simulink model "CK"  (R2023a)
settings: Solver=ode45  StartTime=0.0  StopTime=1000  RelTol=1e-3
values from neighbouring files (symbols this model uses):
  a0 = 0.01    [script.m]
  a1 = 5    [script.m]
  a2 = 10    [script.m]
  Alpha = 1    [script.m]
  b0 = 0.025    [script.m]
  b1 = 0.25    [script.m]
  b2 = 1    [script.m]
  c0 = 0.5    [script.m]
  c1 = 5    [script.m]
  Cyt = 1    [script.m]
  d1 = 1    [script.m]
  k1 = 0.025    [script.m]
  K1 = 1    [script.m]
  K2 = 1    [script.m]
  k2 = 0.5    [script.m]
  Kh1 = 5    [script.m]
  Kh2 = 5    [script.m]
  n = 2    [script.m]
  r1 = 0.025    [script.m]
  r2 = 0.025    [script.m]
  r3 = 0.025    [script.m]
  r4 = 0.025    [script.m]
  V1 = 1    [script.m]
  Vh1 = 2    [script.m]
settings Model: Creator=mosuk  LastModifiedBy=mosuk
settings DataIOCC: ReturnWorkspaceOutputs=off

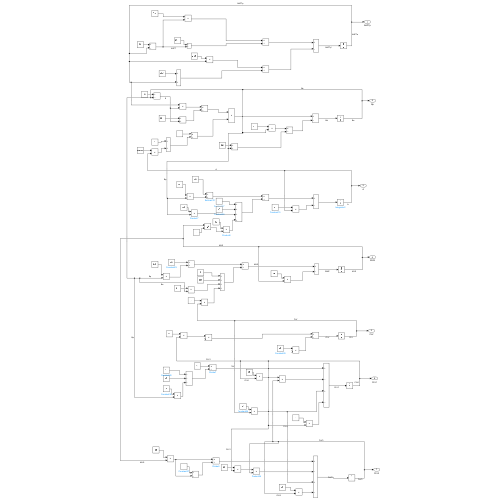
[thumbnail: Simulink's stored preview of the top-level diagram]
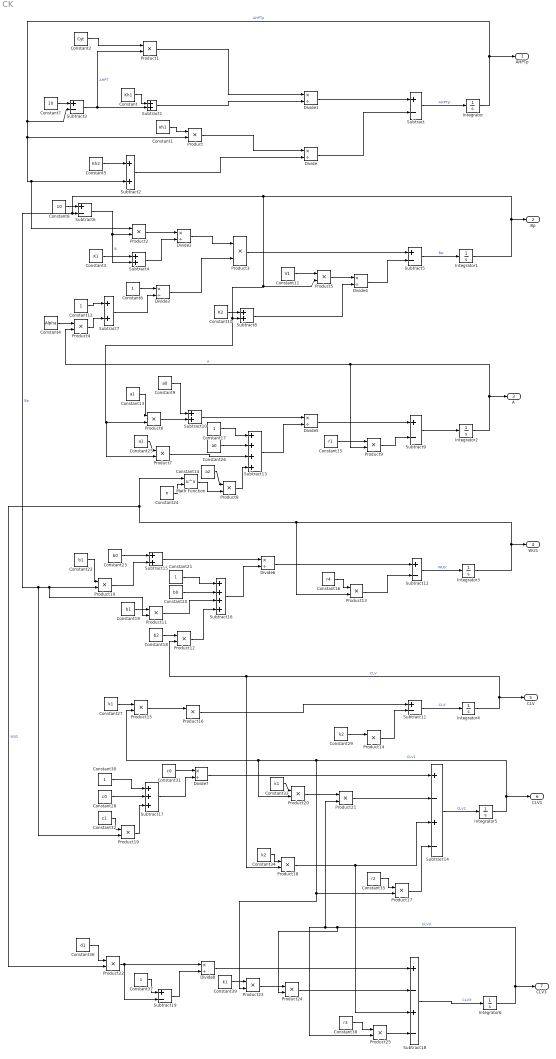
== system CK ==
  Constant : Constant  Value=Kh1
  Constant1 : Constant  Value=Vh1
  Constant10 : Constant  Value=K2
  Constant11 : Constant  Value=V1
  Constant{6,12,17,21,30,37} (6 alike) : Constant
  Constant13 : Constant  Value=a1
  Constant14 : Constant  Value=a2
  Constant15 : Constant  Value=r1
  Constant16 : Constant  Value=r4
  Constant18 : Constant  Value=b2
  Constant19 : Constant  Value=b1
  Constant2 : Constant  Value=Cyt
  Constant20 : Constant  Value=b0
  Constant22 : Constant  Value=b1
  Constant23 : Constant  Value=b0
  Constant24 : Constant  Value=n
  Constant25 : Constant  Value=a1
  Constant26 : Constant  Value=a0
  Constant27 : Constant  Value=k1
  Constant28 : Constant  Value=c0
  Constant29 : Constant  Value=k2
  Constant3 : Constant  Value=K1
  Constant31 : Constant  Value=c0
  Constant32 : Constant  Value=c1
  Constant33 : Constant  Value=k1
  Constant34 : Constant  Value=k2
  Constant35 : Constant  Value=r2
  Constant36 : Constant  Value=d1
  Constant38 : Constant  Value=r3
  Constant39 : Constant  Value=k1
  Constant4 : Constant  Value=Alpha
  Constant5 : Constant  Value=Kh2
  Constant7 : Constant  Value=10
  Constant8 : Constant  Value=10
  Constant9 : Constant  Value=a0
  Divide{,1..8} (9 alike) : Product  Inputs=*/
  Integrator{,1..6} (7 alike) : Integrator
  Math Function : Math  Operator=pow
  Product{,1..25} (26 alike) : Product
  Subtract{,3,5..6,9,11..12,19} (8 alike) : Sum  Inputs=+-
  Subtract{1..2,4,7..8,10,15} (7 alike) : Sum
  Subtract13 : Sum  Inputs=++++
  Subtract14 : Sum  Inputs=+-+-
  Subtract16 : Sum  Inputs=++++
  Subtract17 : Sum  Inputs=+++
  Subtract18 : Sum  Inputs=+-+-
  AHPTp : Outport
  Bp : Outport  Port=2
  A : Outport  Port=3
  WUS : Outport  Port=4
  CLV : Outport  Port=5
  CLV1 : Outport  Port=6
  CLV3 : Outport  Port=7
  wires:
  Integrator/1 -> AHPTp/1, Subtract3/2, Product/2, Product2/1, Subtract2/2  "AHPTp"
  Subtract/1 -> Integrator/1  "AHPTp'"
  Constant/1 -> Subtract1/1
  Constant5/1 -> Subtract2/1
  Subtract2/1 -> Divide/2
  Constant1/1 -> Product/1
  Product/1 -> Divide/1
  Divide/1 -> Subtract/2
  Constant7/1 -> Subtract3/1
  Subtract3/1 -> Product1/2, Subtract1/2  "AHPT"
  Subtract1/1 -> Divide1/2
  Constant2/1 -> Product1/1
  Product1/1 -> Divide1/1
  Divide1/1 -> Subtract/1
  Integrator1/1 -> Bp/1, Product5/2, Product7/2, Product6/2, Subtract8/2, Product19/2, Product11/2, Product10/2, Subtract6/2  "Bp"
  Integrator2/1 -> Product9/2, Product4/2, A/1  "A"
  Constant3/1 -> Subtract4/1
  Constant8/1 -> Subtract6/1
  Subtract6/1 -> Subtract4/2, Product2/2  "B"
  Product2/1 -> Divide2/1
  Subtract4/1 -> Divide2/2
  Divide2/1 -> Product3/1
  Constant6/1 -> Divide3/1
  Constant4/1 -> Product4/1
  Product4/1 -> Subtract7/2
  Constant12/1 -> Subtract7/1
  Subtract7/1 -> Divide3/2
  Divide3/1 -> Product3/2
  Product3/1 -> Subtract5/1
  Constant10/1 -> Subtract8/1
  Constant11/1 -> Product5/1
  Product5/1 -> Divide4/1
  Subtract8/1 -> Divide4/2
  Divide4/1 -> Subtract5/2
  Subtract5/1 -> Integrator1/1  "Bp'"
  Subtract9/1 -> Integrator2/1
  Constant13/1 -> Product6/1
  Product6/1 -> Subtract10/2
  Constant9/1 -> Subtract10/1
  Subtract10/1 -> Divide5/1
  Constant17/1 -> Subtract13/1
  Constant26/1 -> Subtract13/2
  Constant25/1 -> Product7/1
  Product7/1 -> Subtract13/3
  Constant24/1 -> Math Function/2
  Integrator3/1 -> WUS/1, Product13/2, Product22/2, Math Function/1  "WUS"
  Subtract12/1 -> Integrator3/1  "WUS'"
  Math Function/1 -> Product8/2
  Constant14/1 -> Product8/1
  Product8/1 -> Subtract13/4
  Subtract13/1 -> Divide5/2
  Divide5/1 -> Subtract9/1
  Constant15/1 -> Product9/1
  Product9/1 -> Subtract9/2
  Constant22/1 -> Product10/1
  Constant23/1 -> Subtract15/1
  Product10/1 -> Subtract15/2
  Subtract15/1 -> Divide6/1
  Constant21/1 -> Subtract16/1
  Constant20/1 -> Subtract16/2
  Constant19/1 -> Product11/1
  Product11/1 -> Subtract16/3
  Subtract11/1 -> Integrator4/1  "CLV'"
  Integrator4/1 -> Product12/2, Product18/2, CLV/1  "CLV"
  Constant18/1 -> Product12/1
  Product12/1 -> Subtract16/4
  Subtract16/1 -> Divide6/2
  Divide6/1 -> Subtract12/1
  Constant16/1 -> Product13/1
  Product13/1 -> Subtract12/2
  Constant29/1 -> Product14/1
  Constant27/1 -> Product15/1
  Product15/1 -> Product16/1
  Product16/1 -> Subtract11/1
  Product14/1 -> Subtract11/2
  Integrator5/1 -> CLV1/1, Product23/2, Product17/2, Product20/2, Product15/2  "CLV1"
  Subtract14/1 -> Integrator5/1  "CLV1'"
  Constant35/1 -> Product17/1
  Product17/1 -> Subtract14/4
  Constant34/1 -> Product18/1
  Product18/1 -> Subtract18/3, Subtract14/3
  Constant30/1 -> Subtract17/1
  Constant28/1 -> Subtract17/2
  Constant32/1 -> Product19/1
  Product19/1 -> Subtract17/3
  Constant31/1 -> Divide7/1
  Subtract17/1 -> Divide7/2
  Divide7/1 -> Subtract14/1
  Constant33/1 -> Product20/1
  Product20/1 -> Product21/1
  Integrator6/1 -> Product25/2, Product21/2, Product24/2, CLV3/1  "CLV3"
  Subtract18/1 -> Integrator6/1  "CLV3'"
  Constant36/1 -> Product22/1
  Product22/1 -> Subtract19/2, Divide8/1
  Constant37/1 -> Subtract19/1
  Subtract19/1 -> Divide8/2
  Divide8/1 -> Subtract18/1
  Product21/1 -> Subtract14/2
  Constant39/1 -> Product23/1
  Product23/1 -> Product24/1
  Product24/1 -> Subtract18/2
  Constant38/1 -> Product25/1
  Product25/1 -> Subtract18/4
